simulink model "practical_and_ideal_transformer"  (R2014b)
settings: Solver=ode23tb  StartTime=0.0  StopTime=0.2  MaxStep=1e-4  RelTol=1e-3
libraries: powerlib x9, powerlib_meascontrol x6
settings Model: Creator=Amr Saleh  LastModifiedBy=Amr Saleh

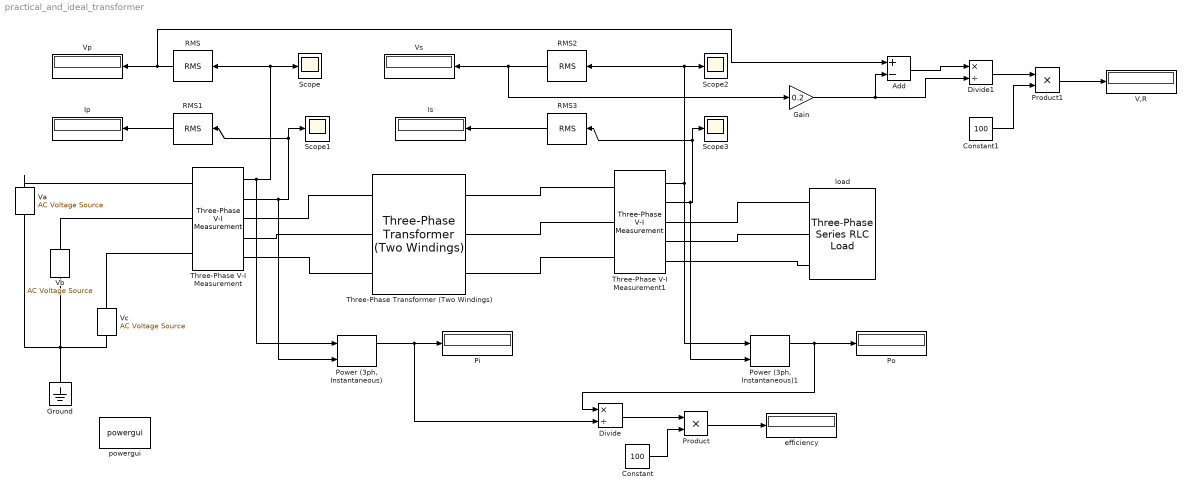
== system practical_and_ideal_transformer ==
  Add : Sum  Inputs=+-
  Constant : Constant  Value=100
  Constant1 : Constant  Value=100
  Divide : Product  Inputs=*/
  Divide1 : Product  Inputs=*/
  Gain : Gain  Gain=0.2
  Ground : powerlib/Elements/Ground  LConnTagsString=a
  Ip : Display
  Is : Display
  Pi : Display
  Po : Display
  "Power (3ph, Instantaneous)" : powerlib_meascontrol/Measurements/Power (3ph, Instantaneous)
  "Power (3ph, Instantaneous)1" : powerlib_meascontrol/Measurements/Power (3ph, Instantaneous)
  Product : Product
  Product1 : Product
  RMS{,1..3} (4 alike) : powerlib_meascontrol/Measurements/RMS  TrueRMS=off  Freq=50  RMSInit=0  Ts=0
  Scope{,1..3} (4 alike) : Scope
      Scope2 settings: SaveName=ScopeData2
      Scope3 settings: SaveName=ScopeData3
  Three-Phase Transformer (Two Windings) : powerlib/Elements/Three-Phase Transformer (Two Windings)  Winding1Connection=Y  UNITS=SI  NominalPower=[ 2000e3 , 50 ]  Winding1=[6.6e3 0.5 8.27e-3]  Winding2Connection=Y  Winding2=[33e3 4.3 0.069]  SetSaturation=off  Rm=10000  Lm=500  Saturation=[0 0;0.59382 20.584;247.42 26.073]  Hysteresis=off  DataFile='hysteresis'  SetInitialFlux=off  InitialFluxes=[13.723 -13.723 12.007]  Measurements=None  MoreParameters=off  BreakLoop=off  DataType=on  TransfoNumber=1
  Three-Phase V-I Measurement : powerlib/Measurements/Three-Phase V-I Measurement  VoltageMeasurement=phase-to-ground  SetLabelV=off  LabelV=Vabc  Vpu=off  VpuLL=off  CurrentMeasurement=yes  SetLabelI=off  LabelI=Iabc  Ipu=off  Pbase=100e6  Vbase=500e3  OutputType=Complex  PhasorSimulation=off  PSBequivalent=0
  Three-Phase V-I Measurement1 : powerlib/Measurements/Three-Phase V-I Measurement  VoltageMeasurement=phase-to-ground  SetLabelV=off  LabelV=Vabc  Vpu=off  VpuLL=off  CurrentMeasurement=yes  SetLabelI=off  LabelI=Iabc  Ipu=off  Pbase=100e6  Vbase=500e3  OutputType=Complex  PhasorSimulation=off  PSBequivalent=0
  V,R : Display
  Va : powerlib/Electrical Sources/AC Voltage Source  Amplitude=6.6*1000*sqrt(2)/sqrt(3)  Phase=0  Frequency=50  SampleTime=0  Measurements=None
  Vb : powerlib/Electrical Sources/AC Voltage Source  Amplitude=6.6*1000*sqrt(2)/sqrt(3)  Phase=-120  Frequency=50  SampleTime=0  Measurements=None
  Vc : powerlib/Electrical Sources/AC Voltage Source  Amplitude=6.6*1000*sqrt(2)/sqrt(3)  Phase=120  Frequency=50  SampleTime=0  Measurements=None
  Vp : Display
  Vs : Display
  efficiency : Display
  load : powerlib/Elements/Three-Phase Series RLC Load  LConnTagsString=A|B|C  Configuration=Y (grounded)  NominalVoltage=33e3  NominalFrequency=50  ActivePower=1600e3  InductivePower=1200e3  CapacitivePower=0  Measurements=None  LoadType=constant Z
  powergui : powerlib/powergui  Priority=1  SimulationMode=Continuous  SolverType=Tustin/Backward Euler (TBE)  SampleTime=50e-6  frequency=60  SPID=off  DisableSnubberDevices=off  DisableRonSwitches=off  DisableVfSwitches=off  SwTol=0  DisplayEquations=off  Interpol=off  methode=off  Ts=100  frequencyindice=50  Pbase=100e6  ErrMax=1e-4  Iterations=50  UnitsV=kV  UnitsW=MW  FunctionMessages=off  echomessages=off  HookPort=off  EnableUseOfTLC=off  x0status=blocks  RestoreLinks=warning  ResistiveCurrentMeasurement=off  Frange=[0:2:500]  Ylog=off  Xlog=on  ShowGrid=off  save=off  variable=ZData  structure=0  ZoomFFT=off  StartTime=0.0  cycles=1  DisplayStyle=1  fundamental=60  FreqAxis=off  MaxFrequency=1000  frequencyindicesteady=1  RmsSteady=1  display=off
  wires:
  Three-Phase V-I Measurement/1 -> "Power (3ph, Instantaneous)"/1, Scope/1, RMS/1
  Three-Phase V-I Measurement/2 -> Scope1/1, RMS1/1, "Power (3ph, Instantaneous)"/2
  RMS/1 -> Add/1, Vp/1
  RMS1/1 -> Ip/1
  Three-Phase V-I Measurement1/1 -> "Power (3ph, Instantaneous)1"/1, RMS2/1, Scope2/1
  Three-Phase V-I Measurement1/2 -> "Power (3ph, Instantaneous)1"/2, Scope3/1, RMS3/1
  RMS2/1 -> Gain/1, Vs/1
  RMS3/1 -> Is/1
  "Power (3ph, Instantaneous)"/1 -> Divide/2, Pi/1
  "Power (3ph, Instantaneous)1"/1 -> Divide/1, Po/1
  Divide/1 -> Product/1
  Constant/1 -> Product/2
  Product/1 -> efficiency/1
  Gain/1 -> Divide1/2, Add/2
  Add/1 -> Divide1/1
  Divide1/1 -> Product1/1
  Constant1/1 -> Product1/2
  Product1/1 -> V,R/1
  connections:
  Vc/LConn1 -- Ground/LConn1 -- Va/LConn1 -- Vb/LConn1
  Va/RConn1 -- Three-Phase V-I Measurement/LConn1
  Three-Phase V-I Measurement/LConn2 -- Vb/RConn1
  Vc/RConn1 -- Three-Phase V-I Measurement/LConn3
  Three-Phase V-I Measurement/RConn1 -- Three-Phase Transformer (Two Windings)/LConn1
  Three-Phase V-I Measurement/RConn2 -- Three-Phase Transformer (Two Windings)/LConn2
  Three-Phase V-I Measurement/RConn3 -- Three-Phase Transformer (Two Windings)/LConn3
  Three-Phase Transformer (Two Windings)/RConn1 -- Three-Phase V-I Measurement1/LConn1
  Three-Phase Transformer (Two Windings)/RConn2 -- Three-Phase V-I Measurement1/LConn2
  Three-Phase Transformer (Two Windings)/RConn3 -- Three-Phase V-I Measurement1/LConn3
  Three-Phase V-I Measurement1/RConn1 -- load/LConn1
  Three-Phase V-I Measurement1/RConn2 -- load/LConn2
  Three-Phase V-I Measurement1/RConn3 -- load/LConn3
